simulink model "DT"  (R2021b)
settings: Solver=VariableStepAuto  StartTime=0.0  StopTime=120*sampleTs  MaxStep=sampleTs*0.1  RelTol=1e-3
model workspace (MAT data in the model file):
  A = [2.10254727061  -1.22446410783  0.12191683722; 1  0  0; 0  1  0]
  B = [1; 0; 0]
  C = [0.00238202414411 0.00238202414411 0]
  D = 0
  F = 0.001
  G2_den = [1 981.079695856 28207.066422 -1.77414671021e-06]
  G2_num = [0 0.252050742588 2193.29302906 5229417.83287]
  I = 0
  Kd = 0.066162109375
  Ki = 0
  Kp = 10.2124023438
  P = 10.5859375
  PD = [5420 41]
  reference = 40
  reference0 = 30
  sampleTs = 0.001
libraries: slpidlib x1
settings Model: Creator=mahdi  LastModifiedBy=mahdi

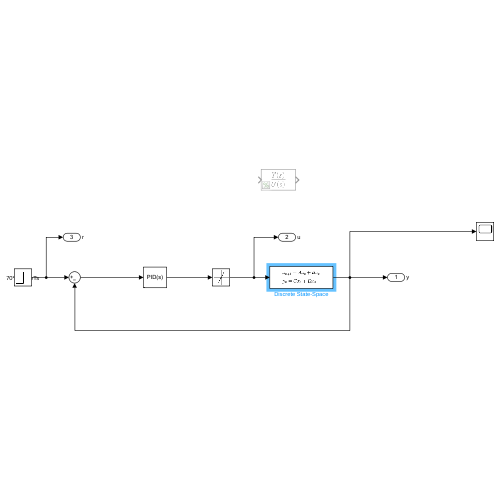
[thumbnail: Simulink's stored preview of the top-level diagram]
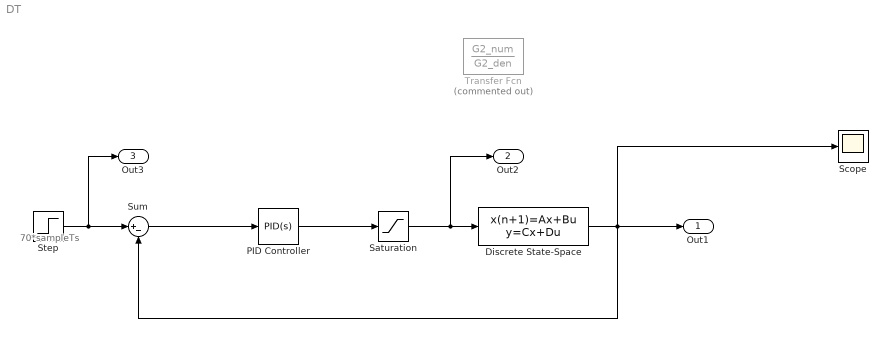
== system DT ==
  note: 70*sampleTs
  Discrete State-Space : DiscreteStateSpace  A=A  B=B  C=C  D=D  InitialCondition=reference0  SampleTime=sampleTs
  PID Controller : slpidlib/PID Controller  Controller=PID  Form=Parallel  TimeDomain=Continuous-time  UseExternalTs=off  SampleTime=-1  IntegratorMethod=Forward Euler  FilterMethod=Forward Euler  ControllerParametersSource=internal  P=P  I=I  D=D  UseFilter=on  N=1/F  TunerSelectOption=Transfer Function Based (PID Tuner App)  InitialConditionSource=internal  InitialConditionForIntegrator=0  InitialConditionForFilter=0  DifferentiatorICPrevScaledInput=0  ExternalReset=none  TrackingMode=off  Kt=1  LimitOutput=off  SatLimitsSource=internal  UpperSaturationLimit=inf  LowerSaturationLimit=-inf  LinearizeAsGain=on  AntiWindupMode=none  Kb=1  POutMin=[]  POutMax=[]  IOutMin=[]  IOutMax=[]  DOutMin=[]  DOutMax=[]  NOutMin=[]  NOutMax=[]  SumOutMin=[]  SumOutMax=[]  SaturationOutMin=[]  SaturationOutMax=[]  PParamMin=[]  PParamMax=[]  IParamMin=[]  IParamMax=[]  DParamMin=[]  DParamMax=[]  NParamMin=[]  NParamMax=[]  KbParamMin=[]  KbParamMax=[]  KtParamMin=[]  KtParamMax=[]  KbOutMin=[]  KbOutMax=[]  KtOutMin=[]  KtOutMax=[]  IntegratorOutMin=[]  IntegratorOutMax=[]  FilterOutMin=[]  FilterOutMax=[]  SumI1OutMin=[]  SumI1OutMax=[]  SumI2OutMin=[]  SumI2OutMax=[]  SumI3OutMin=[]  SumI3OutMax=[]  SumI4OutMin=[]  SumI4OutMax=[]  SumDOutMin=[]  SumDOutMax=[]  DifferentiatorOutMin=[]  DifferentiatorOutMax=[]  FilterDiffOutCoefMin=[]  FilterDiffOutCoefMax=[]  ReciprocalOutMin=[]  ReciprocalOutMax=[]  SumDenOutMin=[]  SumDenOutMax=[]  SumNumOutMin=[]  SumNumOutMax=[]  DivideOutMin=[]  DivideOutMax=[]  UdiffTsProdOutMin=[]  UdiffTsProdOutMax=[]  NTsProdOutMin=[]  NTsProdOutMax=[]  UintegralTsProdOutMin=[]  UintegralTsProdOutMax=[]  UngainTsProdOutMin=[]  UngainTsProdOutMax=[]  FilterDenConstantOutDataTypeStr=Inherit: Inherit via back propagation  FilterDenConstantOutMin=[]  FilterDenConstantOutMax=[]  PCopyOutDataTypeStr=Inherit: Inherit via back propagation  PCopyOutMin=[]  PCopyOutMax=[]  NCopyOutDataTypeStr=Inherit: Inherit via back propagation  NCopyOutMin=[]  NCopyOutMax=[]  IntegratorContinuousStateAttributes=''  IntegratorStateMustResolveToSignalObject=off  IntegratorRTWStateStorageClass=Auto  FilterContinuousStateAttributes=''  FilterStateMustResolveToSignalObject=off  FilterRTWStateStorageClass=Auto  ParallelPVariant=InternalParameters  IdealPVariant=Disabled  IVariant=InternalParameters  DVariant=InternalParameters  IntegratorVariant=Continuous  SatVariant=Disabled  AWVariant=Passthrough  PCopyVariant=Disabled  TRVariant=Disabled  FdbkBlocksVariant=Forward  IdealPFdbkVariant=Disabled  SatFdbkVariant=Disabled  DerivativeFilterVariant=ContFilter  NVariant=InternalParameters  NCopyVariant=Disabled  FilterICVariant=InternalICsFilter  IntegratorICVariant=InternalICs  ExternalResetVariant=Disabled  TRSumVariant=Passthrough  SumFdbkVariant=Disabled  SumVariant=Sum_PID  TsampFilterVariant=InternalTs  TsampNgainVariant=Passthrough  TsampIntegralVariant=Passthrough  ExternalSaturationOutDataTypeStr=Inherit: Same as second input
  Saturation : Saturate  UpperLimit=7  LowerLimit=-7  ZeroCross=off
  Scope : Scope
  Step : Step  Time=50*sampleTs  Before=reference0  After=reference  SampleTime=sampleTs
  Sum : Sum  Inputs=|+-
  Transfer Fcn : TransferFcn  Commented=on  Numerator=G2_num  Denominator=G2_den
  Out1 : Outport  SignalName=y
  Out2 : Outport  Port=2  SignalName=u
  Out3 : Outport  Port=3  SignalName=r
  wires:
  PID Controller/1 -> Saturation/1
  Saturation/1 -> Out2/1, Discrete State-Space/1
  Step/1 -> Out3/1, Sum/1
  Sum/1 -> PID Controller/1
  Discrete State-Space/1 -> Scope/1, Out1/1, Sum/2
